simulink model "ddv_ssv_control"  (R2024a)
settings: Solver=VariableStepAuto  StartTime=0.0  StopTime=60  RelTol=1e-3
settings Model: Creator=giuli  LastModifiedBy=MARTENAG

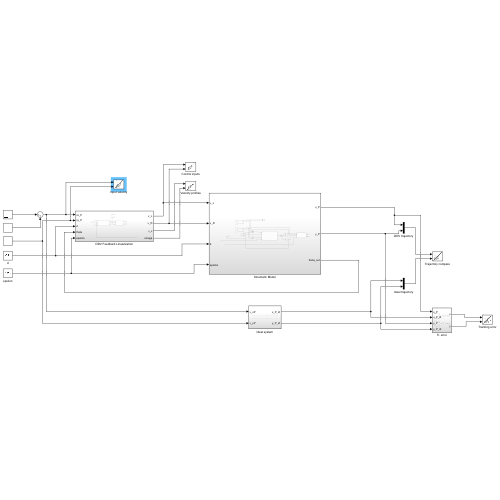
[thumbnail: Simulink's stored preview of the top-level diagram]
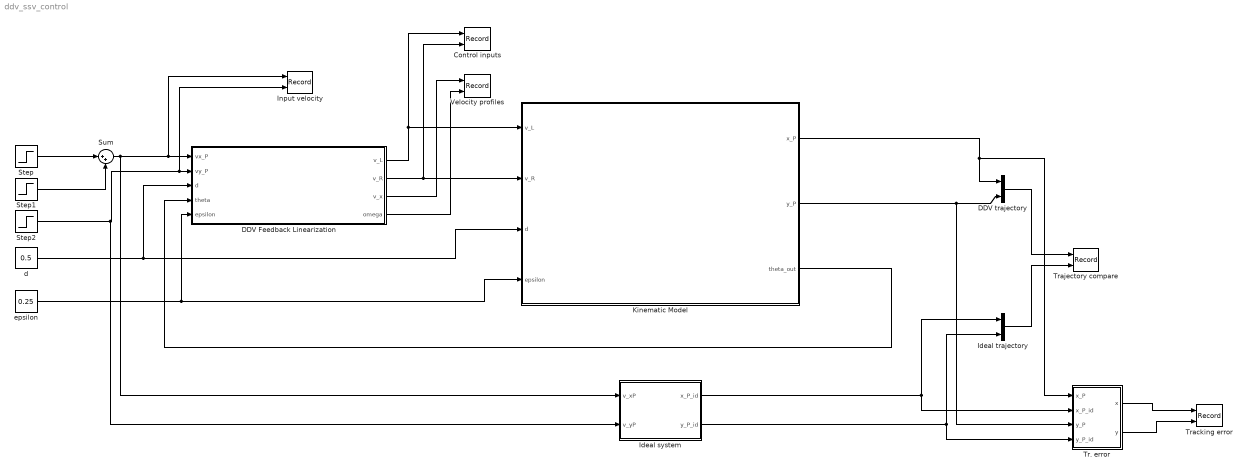
== system ddv_ssv_control ==
  Control inputs : Record  FileSettingsInternal="{\"entries\":[{\"content\":{\"excelSettings\":{\"content\":{},\"type\":\"Streamout.ExcelSettings\"}},\"type\":\"Streamout.FileSettingStorage\",\"uuid\":\"\"}],\"packageUris\":[\"http:\\/\\/schema.mathworks.com\\/mf0\\/streamout_blocks\\/R2020a\"],\"version\":\"1.0\"}"  Layout=[1 1]  SignalsInternal="{\"entries\":[{\"content\":{\"signals\":[{\"content\":{\"blockPath\":[],\"dimensions\":[1],\"domain\":\"\",\"lineColor\":\"#ff6929\",\"lineWidth\":2,\"port\":1,\"sid\":[\"\"],\"signalID\":1,\"signalName\":\"DDV Feedback Linearization:1\"},\"type\":\"RecordBlkView.Signal\",\"uuid\":\"\"},{\"content\":{\"blockPath\":[],\"dimensions\":[1],\"domain\":\"\",\"lineColor\":\"#b746ff\",\"lineWidth\":2,\"port\":2,\"sid\":[\"\"],\"signalID\":2,\"signalName\":\"DDV Feedback Linearization:2\"},\"type\":\"RecordBlkView.Signal\",\"uuid\":\"\"}]},\"type\":\"RecordBlkView.InputSignals\",\"uuid\":\"\"}],\"packageUris\":[\"http:\\/\\/schema.mathworks.com\\/mf0\\/streamout_blocks\\/R2020a\"],\"version\":\"1.0\"}"  VisualizationBindings="{\"sparklinesplugin\":{\"info\":[{\"bindingParametersList\":[],\"subplotID\":1}]}}"  CompatibilityTag=XY
  DDV Feedback Linearization : Subsystem
  DDV trajectory : Mux  Inputs=2
  Ideal system : Subsystem
  Ideal trajectory : Mux  Inputs=2
  Input velocity : Record  FileSettingsInternal="{\"entries\":[{\"content\":{\"excelSettings\":{\"content\":{},\"type\":\"Streamout.ExcelSettings\"}},\"type\":\"Streamout.FileSettingStorage\",\"uuid\":\"\"}],\"packageUris\":[\"http:\\/\\/schema.mathworks.com\\/mf0\\/streamout_blocks\\/R2020a\"],\"version\":\"1.0\"}"  Layout=[1 1]  SignalsInternal="{\"entries\":[{\"content\":{\"signals\":[{\"content\":{\"blockPath\":[],\"dimensions\":[1],\"domain\":\"\",\"lineColor\":\"#a2142f\",\"plots\":[ 1 ],\"port\":1,\"sid\":[\"\"],\"signalID\":1,\"signalName\":\"Sum\"},\"type\":\"RecordBlkView.Signal\",\"uuid\":\"\"},{\"content\":{\"blockPath\":[],\"dimensions\":[1],\"domain\":\"\",\"lineColor\":\"#139fff\",\"plots\":[ 1 ],\"port\":2,\"sid\":[\"\"],\"signalID\":2,\"signalName\":\"Step2\"},\"type\":\"RecordBlkView.Signal\",\"uuid\":\"\"}]},\"type\":\"RecordBlkView.InputSignals\",\"uuid\":\"\"}],\"packageUris\":[\"http:\\/\\/schema.mathworks.com\\/mf0\\/streamout_blocks\\/R2020a\"],\"version\":\"1.0\"}"  VisualizationBindings="{\"sparklinesplugin\":{\"info\":[{\"bindingParametersList\":[],\"subplotID\":1}]}}"  CompatibilityTag=XY
  Kinematic Model : Subsystem
  Step : Step  SampleTime=0
  Step1 : Step  Time=5  SampleTime=0
  Step2 : Step  Time=10  SampleTime=0
  Sum : Sum  Inputs=|++
  Tr. error : Subsystem
  Tracking error : Record  FileSettingsInternal="{\"entries\":[{\"content\":{\"excelSettings\":{\"content\":{},\"type\":\"Streamout.ExcelSettings\"}},\"type\":\"Streamout.FileSettingStorage\",\"uuid\":\"\"}],\"packageUris\":[\"http:\\/\\/schema.mathworks.com\\/mf0\\/streamout_blocks\\/R2020a\"],\"version\":\"1.0\"}"  Layout=[1 1]  SignalsInternal="{\"entries\":[{\"content\":{\"signals\":[{\"content\":{\"blockPath\":[],\"dimensions\":[1],\"domain\":\"\",\"lineColor\":\"#fe330a\",\"lineWidth\":2,\"port\":1,\"sid\":[\"\"],\"signalID\":1,\"signalName\":\"Tr. error:1\"},\"type\":\"RecordBlkView.Signal\",\"uuid\":\"\"},{\"content\":{\"blockPath\":[],\"dimensions\":[1],\"domain\":\"\",\"lineColor\":\"#22b573\",\"lineWidth\":2,\"port\":2,\"sid\":[\"\"],\"signalID\":2,\"signalName\":\"Tr. error:2\"},\"type\":\"RecordBlkView.Signal\",\"uuid\":\"\"}]},\"type\":\"RecordBlkView.InputSignals\",\"uuid\":\"\"}],\"packageUris\":[\"http:\\/\\/schema.mathworks.com\\/mf0\\/streamout_blocks\\/R2020a\"],\"version\":\"1.0\"}"  CompatibilityTag=XY
  Trajectory compare : Record  FileSettingsInternal="{\"entries\":[{\"content\":{\"excelSettings\":{\"content\":{},\"type\":\"Streamout.ExcelSettings\"}},\"type\":\"Streamout.FileSettingStorage\",\"uuid\":\"\"}],\"packageUris\":[\"http:\\/\\/schema.mathworks.com\\/mf0\\/streamout_blocks\\/R2020a\"],\"version\":\"1.0\"}"  Layout=[1 1]  SignalsInternal="{\"entries\":[{\"content\":{\"signals\":[{\"content\":{\"blockPath\":[],\"dimensions\":[2],\"domain\":\"\",\"hasChildren\":true,\"lineColor\":\"#0072bd\",\"lineWidth\":2,\"port\":1,\"sid\":[\"\"],\"signalID\":1,\"signalName\":\"DDV trajectory\"},\"type\":\"RecordBlkView.Signal\",\"uuid\":\"\"},{\"content\":{\"blockPath\":[],\"channel\":[1],\"dimensions\":[2],\"domain\":\"\",\"lineColor\":\"#d95319\",\"lineWidth\":2,\"parentID\":1,\"port\":1,\"sid\":[\"\"],\"signalID\":2,\"signalName\":\"DDV trajectory\"},\"type\":\"RecordBlkView.Signal\",\"uuid\":\"\"},{\"content\":{\"blockPath\":[],\"dimensions\":[2],\"domain\":\"\",\"hasChildren\":true,\"lineColor\":\"#edb120\",\"lineWidth\":2,\"port\":2,\"sid\":[\"\"],\"signalID\":3,\"signalName\":\"Ideal trajectory\"},\"type\":\"RecordBlkView.Signal\",\"uuid\":\"\"},{\"content\":{\"blockPath\":[],\"channel\":[1],\"dimensions\":[2],\"domain\":\"\",\"lineColor\":\"#7e2f8e\",\"lineWidth\":2,\"parentID\":3,\"port\":2,\"sid\":[\"\"],\"signalID\":4,\"signalName\":\"Ideal trajectory\"},\"type\":\"RecordBlkView.Signal\",\"uuid\":\"\"},{\"content\":{\"blockPath\":[],\"channel\":[2],\"dimensions\":[2],\"domain\":\"\",\"lineColor\":\"#ff6929\",\"lineWidth\":2,\"parentID\":1,\"port\":1,\"sid\":[\"\"],\"signalID\":5,\"signalName\":\"DDV trajectory\"},\"type\":\"RecordBlkView.Signal\",\"uuid\":\"\"},{\"content\":{\"blockPath\":[],\"channel\":[2],\"dimensions\":[2],\"domain\":\"\",\"lineColor\":\"#b746ff\",\"lineWidth\":2,\"parentID\":3,\"port\":2,\"sid\":[\"\"],\"signalID\":6,\"signalName\":\"Ideal trajectory\"},\"type\":\"RecordBlkView.Signal\",\"uuid\":\"\"}]},\"type\":\"RecordBlkView.InputSignals\",\"uuid\":\"\"}],\"packageUris\":[\"http:\\/\\/schema.mathworks.com\\/mf0\\/streamout_blocks\\/R2020a\"],\"version\":\"1.0\"}"  VisualizationBindings="{\"xyplotplugin\":{\"info\":[{\"series\":[],\"subplotID\":1}]}}"  CompatibilityTag=XY
  Velocity profiles : Record  FileSettingsInternal="{\"entries\":[{\"content\":{\"excelSettings\":{\"content\":{},\"type\":\"Streamout.ExcelSettings\"}},\"type\":\"Streamout.FileSettingStorage\",\"uuid\":\"\"}],\"packageUris\":[\"http:\\/\\/schema.mathworks.com\\/mf0\\/streamout_blocks\\/R2020a\"],\"version\":\"1.0\"}"  Layout=[1 1]  SignalsInternal="{\"entries\":[{\"content\":{\"signals\":[{\"content\":{\"blockPath\":[],\"dimensions\":[1],\"domain\":\"\",\"lineColor\":\"#77ac30\",\"lineWidth\":2,\"port\":1,\"sid\":[\"\"],\"signalID\":1,\"signalName\":\"DDV Feedback Linearization:3\"},\"type\":\"RecordBlkView.Signal\",\"uuid\":\"\"},{\"content\":{\"blockPath\":[],\"dimensions\":[1],\"domain\":\"\",\"lineColor\":\"#4dbeee\",\"lineWidth\":2,\"port\":2,\"sid\":[\"\"],\"signalID\":2,\"signalName\":\"DDV Feedback Linearization:4\"},\"type\":\"RecordBlkView.Signal\",\"uuid\":\"\"}]},\"type\":\"RecordBlkView.InputSignals\",\"uuid\":\"\"}],\"packageUris\":[\"http:\\/\\/schema.mathworks.com\\/mf0\\/streamout_blocks\\/R2020a\"],\"version\":\"1.0\"}"  VisualizationBindings="{\"sparklinesplugin\":{\"info\":[{\"bindingParametersList\":[],\"subplotID\":1}]}}"  CompatibilityTag=XY
  d : Constant  Value=0.5
  epsilon : Constant  Value=0.25
  wires:
  d/1 -> DDV Feedback Linearization/3(d), Kinematic Model/3(d)
  Step/1 -> Sum/1
  Step1/1 -> Sum/2
  epsilon/1 -> DDV Feedback Linearization/5(epsilon), Kinematic Model/4(epsilon)
  DDV trajectory/1 -> Trajectory compare/1
  Ideal trajectory/1 -> Trajectory compare/2
  Kinematic Model/1(x_P) -> DDV trajectory/1, Tr. error/1(x_P)
  Kinematic Model/2(y_P) -> Tr. error/3(y_P), DDV trajectory/2
  DDV Feedback Linearization/1(v_L) -> Control inputs/1, Kinematic Model/1(v_L)
  DDV Feedback Linearization/2(v_R) -> Kinematic Model/2(v_R), Control inputs/2
  Kinematic Model/3(theta_out) -> DDV Feedback Linearization/4(theta)
  Ideal system/1(x_P_id) -> Tr. error/2(x_P_id), Ideal trajectory/1
  Ideal system/2(y_P_id) -> Tr. error/4(y_P_id), Ideal trajectory/2
  Tr. error/1(x) -> Tracking error/1
  Tr. error/2(y) -> Tracking error/2
  DDV Feedback Linearization/3(v_x) -> Velocity profiles/1
  DDV Feedback Linearization/4(omega) -> Velocity profiles/2
  Sum/1 -> Ideal system/1(v_xP), Input velocity/1, DDV Feedback Linearization/1(vx_P)
  Step2/1 -> Ideal system/2(v_yP), Input velocity/2, DDV Feedback Linearization/2(vy_P)

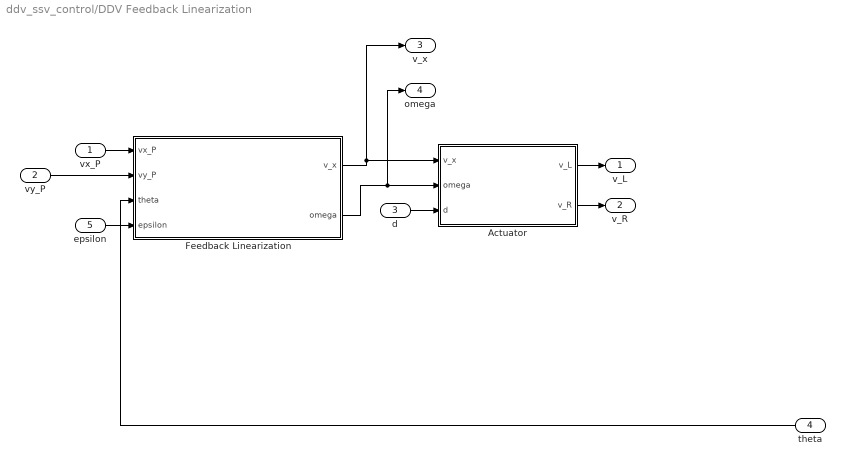
== system ddv_ssv_control/DDV Feedback Linearization ==
  vx_P : Inport
  vy_P : Inport  Port=2
  d : Inport  Port=3
  theta : Inport  Port=4
  epsilon : Inport  Port=5
  Actuator : MATLAB Function  TreatAsAtomicUnit=on
  Feedback Linearization : MATLAB Function  TreatAsAtomicUnit=on
  v_L : Outport
  v_R : Outport  Port=2
  v_x : Outport  Port=3
  omega : Outport  Port=4
  wires:
  vx_P/1 -> Feedback Linearization/1(vx_P)
  Feedback Linearization/2(omega) -> omega/1, Actuator/2(omega)
  Feedback Linearization/1(v_x) -> v_x/1, Actuator/1(v_x)
  d/1 -> Actuator/3(d)
  Actuator/1(v_L) -> v_L/1
  vy_P/1 -> Feedback Linearization/2(vy_P)
  theta/1 -> Feedback Linearization/3(theta)
  Actuator/2(v_R) -> v_R/1
  epsilon/1 -> Feedback Linearization/4(epsilon)

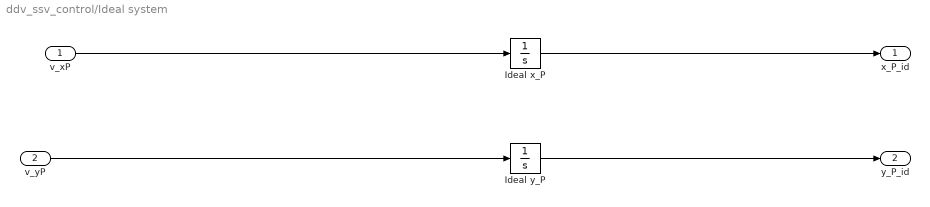
== system ddv_ssv_control/Ideal system ==
  v_xP : Inport
  v_yP : Inport  Port=2
  Ideal x_P : Integrator
  Ideal y_P : Integrator
  x_P_id : Outport
  y_P_id : Outport  Port=2
  wires:
  Ideal x_P/1 -> x_P_id/1
  Ideal y_P/1 -> y_P_id/1
  v_yP/1 -> Ideal y_P/1
  v_xP/1 -> Ideal x_P/1

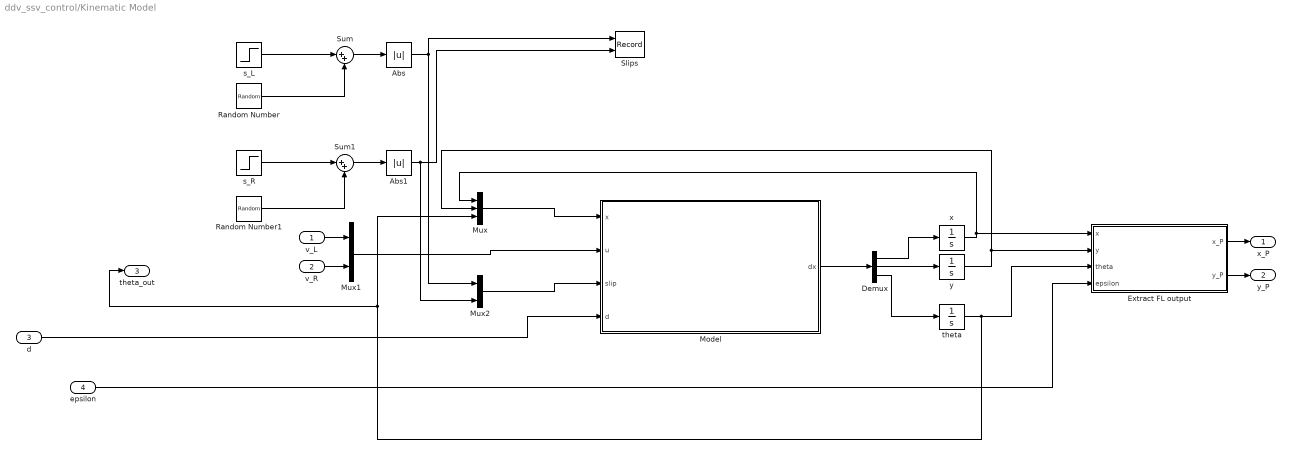
== system ddv_ssv_control/Kinematic Model ==
  v_L : Inport
  v_R : Inport  Port=2
  d : Inport  Port=3
  epsilon : Inport  Port=4
  Abs : Abs  SaturateOnIntegerOverflow=off
  Abs1 : Abs  SaturateOnIntegerOverflow=off
  Demux : Demux  Outputs=3
  Extract FL output : MATLAB Function  TreatAsAtomicUnit=on
  Model : MATLAB Function  TreatAsAtomicUnit=on
  Mux : Mux  Inputs=3
  Mux1 : Mux  Inputs=2
  Mux2 : Mux  Inputs=2
  Random Number : RandomNumber  Mean=0.08  Variance=0.01  SampleTime=0.1
  Random Number1 : RandomNumber  Mean=0.08  Variance=0.01  SampleTime=0.1
  Slips : Record  FileSettingsInternal="{\"entries\":[{\"content\":{\"excelSettings\":{\"content\":{},\"type\":\"Streamout.ExcelSettings\"}},\"type\":\"Streamout.FileSettingStorage\",\"uuid\":\"\"}],\"packageUris\":[\"http:\\/\\/schema.mathworks.com\\/mf0\\/streamout_blocks\\/R2020a\"],\"version\":\"1.0\"}"  Layout=[1 1]  SignalsInternal="{\"entries\":[{\"content\":{\"signals\":[{\"content\":{\"blockPath\":[],\"dimensions\":[1],\"domain\":\"\",\"lineColor\":\"#a2142f\",\"plots\":[ 1 ],\"port\":1,\"sid\":[\"\"],\"signalID\":1,\"signalName\":\"Abs\"},\"type\":\"RecordBlkView.Signal\",\"uuid\":\"\"},{\"content\":{\"blockPath\":[],\"dimensions\":[1],\"domain\":\"\",\"lineColor\":\"#139fff\",\"plots\":[ 1 ],\"port\":2,\"sid\":[\"\"],\"signalID\":2,\"signalName\":\"Abs1\"},\"type\":\"RecordBlkView.Signal\",\"uuid\":\"\"}]},\"type\":\"RecordBlkView.InputSignals\",\"uuid\":\"\"}],\"packageUris\":[\"http:\\/\\/schema.mathworks.com\\/mf0\\/streamout_blocks\\/R2020a\"],\"version\":\"1.0\"}"  VisualizationBindings="{\"sparklinesplugin\":{\"info\":[{\"bindingParametersList\":[],\"subplotID\":1}]}}"  CompatibilityTag=XY
  Sum : Sum  Inputs=|++
  Sum1 : Sum  Inputs=|++
  s_L : Step  Time=6  Before=0.05  After=0.1  SampleTime=0
  s_R : Step  Time=6  Before=0.05  After=0.1  SampleTime=0
  theta : Integrator
  x : Integrator
  y : Integrator
  x_P : Outport
  y_P : Outport  Port=2
  theta_out : Outport  Port=3
  wires:
  Demux/2 -> y/1
  x/1 -> Mux/1, Extract FL output/1(x)
  Mux1/1 -> Model/2(u)
  Mux/1 -> Model/1(x)
  d/1 -> Model/4(d)
  epsilon/1 -> Extract FL output/4(epsilon)
  Model/1(dx) -> Demux/1
  Demux/1 -> x/1
  theta/1 -> Extract FL output/3(theta), theta_out/1, Mux/3
  Mux2/1 -> Model/3(slip)
  Demux/3 -> theta/1
  y/1 -> Extract FL output/2(y), Mux/2
  Extract FL output/1(x_P) -> x_P/1
  v_L/1 -> Mux1/1
  v_R/1 -> Mux1/2
  Extract FL output/2(y_P) -> y_P/1
  s_L/1 -> Sum/1
  Random Number/1 -> Sum/2
  s_R/1 -> Sum1/1
  Random Number1/1 -> Sum1/2
  Sum/1 -> Abs/1
  Abs/1 -> Mux2/1, Slips/1
  Sum1/1 -> Abs1/1
  Abs1/1 -> Slips/2, Mux2/2

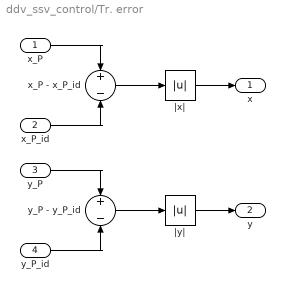
== system ddv_ssv_control/Tr. error ==
  x_P : Inport
  x_P_id : Inport  Port=2
  y_P : Inport  Port=3
  y_P_id : Inport  Port=4
  x_P - x_P_id : Sum  Inputs=+-
  y_P - y_P_id : Sum  Inputs=+-
  |x| : Abs  SaturateOnIntegerOverflow=off
  |y| : Abs  SaturateOnIntegerOverflow=off
  x : Outport
  y : Outport  Port=2
  wires:
  y_P/1 -> y_P - y_P_id/1
  x_P/1 -> x_P - x_P_id/1
  y_P_id/1 -> y_P - y_P_id/2
  x_P_id/1 -> x_P - x_P_id/2
  |y|/1 -> y/1
  x_P - x_P_id/1 -> |x|/1
  y_P - y_P_id/1 -> |y|/1
  |x|/1 -> x/1

== matlab function ddv_ssv_control/DDV Feedback Linearization/Feedback Linearization ==
  data: vx_P input; v_x output; vy_P input; theta input; omega output; epsilon input
function [v_x, omega] = ddv_feedback_linearization(vx_P, vy_P, theta, epsilon)

   v_x = vx_P * cos(theta) + vy_P * sin(theta);
   omega = (-1/epsilon * sin(theta)) * vx_P + (1/epsilon * cos(theta)) * vy_P;
end

== matlab function ddv_ssv_control/Kinematic Model/Model ==
  data: x input size=3; dx output size=3; u input size=2; slip input size=2; d input size=1
function dx = kinematic_model(x, u, slip, d)
% Inputs:
    % x = [x; y; theta] (state vector)
    % u = [v_L; v_R] (control inputs: left and right wheel velocities)
    % slip = [s_L; s_R] (slip coefficients for left and right wheels)
    % d (half the track width)
    
    % Extract slip
    s_L = slip(1);
    s_R = slip(2);

    % Extract state variables
    theta = x(3);

    % Extract control inputs
    v_L = u(1);
    v_R = u(2);
    
    % Kinematic equations
    dx = zeros(3,1);
    dx(1) = ((1-s_R)/2 * cos(theta) * v_R) + ((1-s_L)/2 * cos(theta) * v_L);
    dx(2) = ((1-s_R)/2 * sin(theta) * v_R) + ((1-s_L)/2 * sin(theta) * v_L);
    dx(3) = (1-s_R)/(2*d)*v_R - (1-s_L)/(2*d)*v_L;
end

== matlab function ddv_ssv_control/DDV Feedback Linearization/Actuator ==
  data: v_x input; v_L output; omega input; d input; v_R output
function [v_L, v_R] = actuator(v_x, omega, d)
    v_L = v_x - d*omega;
    v_R = v_x + d*omega;
end

== matlab function ddv_ssv_control/Kinematic Model/Extract FL output ==
  data: x input; x_P output; y input; theta input; epsilon input; y_P output
function [x_P, y_P] = extract_fl_output(x, y, theta, epsilon)
    x_P = x + epsilon*cos(theta);
    y_P = y + epsilon*sin(theta);
end
